simulink model "navigation_filter"  (R2024b)
settings: Solver=FixedStepAuto  StartTime=0.0  StopTime=200.0  FixedStep=ST  RelTol=1e-3
values from neighbouring files (symbols this model uses):
  bias_gyro = [0.02 0.01 0.007]    [sensors.m]    (also in sensors_2.m = [0.2 0.1 0])
  dt = ST    (= 0.01)    [WP_gen.m]
  freq_acc = 50    [sensors.m]    (also in sensors_2.m)
  freq_gyro = 10    [sensors.m]    (also in sensors_2.m)
  freq_UWB = freq_gyro    (= 10)    [sensors.m]    (also in sensors_2.m)
  g = 9.81    [trajectory_gen_cartesian.m]
  N_bases = size(P_bases_ned, 1)    [sensors.m]    (also in sensors_2.m)
  pos_ned = [pos_ned_n pos_ned_e pos_ned_d]    [WP_gen.m]    (also in trajectory_gen_cartesian.m = pos_n_filt)
  Q = 100*diag([q_pos_1, q_pos_2, q_pos_3, q_vel_1, q_vel_2, q_vel_3, q_acc_1,q_acc_2,q_acc_3, q_quat_1, q_quat_2, q_quat_3, q_quat_4, q_omega_1, q_omega_2, q_omega_3, q_bias_1, q_bias_2, q_bias_3])    [sensors.m]    (also in sensors_2.m)
  Q_att = 100*diag([q_roll, q_pitch, q_yaw, q_omega_1, q_omega_2, q_omega_3, q_bias_1, q_bias_2, q_bias_3])    [sensors_2.m]
  quat_c_b = compact(quat_b)    [trajectory_gen_cartesian.m]
  sensor_covariances = [UWB_cov, ACC_cov, MAG_cov, GYRO_cov]    [sensors.m]    (also in sensors_2.m)
  ST = 1/100    (= 0.01)    [WP_gen.m]
  std_dev_accx = 0.02    [sensors.m]    (also in sensors_2.m = 0.01)
  std_dev_accy = 0.02    [sensors.m]    (also in sensors_2.m = 0.01)
  std_dev_accz = 0.02    [sensors.m]    (also in sensors_2.m = 0.01)
  std_dev_gyro1 = 1e-7    (= 1e-07)    [sensors.m]    (also in sensors_2.m = 3e-06)
  std_dev_gyro2 = 1e-7    (= 1e-07)    [sensors.m]    (also in sensors_2.m = 3e-06)
  std_dev_gyro3 = 1e-7    (= 1e-07)    [sensors.m]    (also in sensors_2.m = 3e-06)
  std_dev_magx = 0.03    [sensors.m]    (also in sensors_2.m)
  std_dev_magy = 0.03    [sensors.m]    (also in sensors_2.m)
  std_dev_magz = 0.03    [sensors.m]    (also in sensors_2.m)
  std_dev_UWB1 = 1e-6    (= 1e-06)    [sensors.m]    (also in sensors_2.m)
  Tf = ST    [sensors.m]    (also in sensors_2.m)
  vel_n = vel_n_filt    [trajectory_gen_cartesian.m]
undefined symbols (not defined in the file or in its folder): DiscIntNeverNeededParam
libraries: cstblocks x8, simulink x3, aerolibutil x2
(part 1 of 2)
settings Model: Creator=wolfl  LastModifiedBy=wolfl

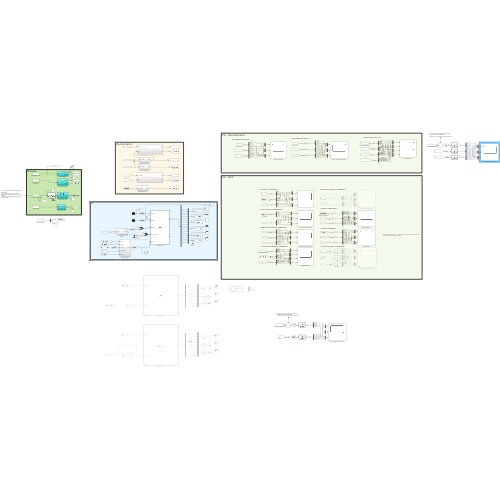
[thumbnail: Simulink's stored preview of the top-level diagram]
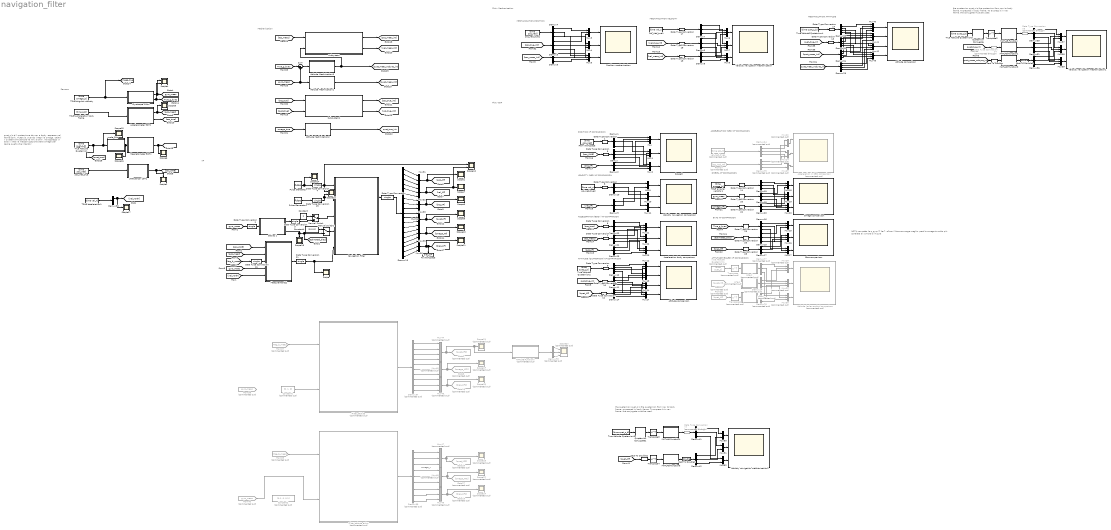
== system navigation_filter ==
  note: omega_x
  note: the quaternion quat_c is the quaternion from nav to
      | body frame, expressed in body frame.
      | To express it in nav frame, the conjugate must be used.
  note: quat_c_b è il quaternione da nav a body, espresso nel frame body.
      | Tuttavia, quando integri la omega, ottieni il quaternione sempre da nav a body, ma espresso in body!!!
      | Vedi la meccanizzazione della omega per capire quello che intendo!
  note: NOTA: se metto le q_gyro = 1e-7, allora il bias converge meglio, però la omega
      | è molto più correlata al rumore di misura
  note: Plot - EKF
  note: KF
  note: Mechanization
  note: Sensors
  note: Plot - Mechanization
  note: MECHANIZATION POSITION
  note: MECHANIZATION VELOCITY
  note: ATTUTUDE (EULER) KF COMPARISON
  note: ATTITUDE (QUATERNION) KF COMPARISON
  note: OMEGA KF COMPARISON
  note: ACCELERATION (BODY) KF COMPARISON
  note: VELOCITY (NED) KF COMPARISON
  note: POSITION KF COMPARISON
  note: BYAS KF COMPARISON
  note: ACCELERATION (NED) KF COMPARISON
  note: MECHANIZATION ATTITUDE
  note: the quaternion quat_c is the quaternion from nav to
      | body frame, expressed in body frame.
      | To express it in nav frame, the conjugate must be used.
  Acceleration body comparison : Scope  NumInputPorts=3
  Acceleration in NED comparison : Scope  Commented=on  NumInputPorts=3
  Accelerometer 50Hz : Subsystem
  Attitude (euler angles) comparison : Scope  Commented=on  NumInputPorts=3
  Attitude Mechnization1 : Subsystem
  Attitude Mechnization2 : Subsystem
  Attitude Mechnization3 : Subsystem
  "Attitude comparison " : Scope  NumInputPorts=4
  "Attitude comparison " : Scope  NumInputPorts=4
  Bias comparison : Scope  NumInputPorts=3
  Cast To Double{,1..3} (4 alike) : DataTypeConversion  OutDataTypeStr=double  SaturateOnIntegerOverflow=off  RndMeth=Floor
  Constant : Constant
  Constant1 : Constant  Commented=on  Value=[0, 1, 0]
  Constant2 : Constant  Commented=on  Value=[0.1, 0, 0.1]
  Constant4 : Constant  Value=[0 0 0]
  Data Type Conversion{,1..23,26,28} (26 alike) : DataTypeConversion  OutDataTypeStr=single  SaturateOnIntegerOverflow=off  RndMeth=Floor
  Data Type Conversion24 : DataTypeConversion  Commented=through  OutDataTypeStr=single  SaturateOnIntegerOverflow=off  RndMeth=Floor
  Data Type Conversion25 : DataTypeConversion  Commented=through  OutDataTypeStr=single  SaturateOnIntegerOverflow=off  RndMeth=Floor
  Data Type Conversion27 : DataTypeConversion  Commented=through  OutDataTypeStr=single  SaturateOnIntegerOverflow=off  RndMeth=Floor
  Demux{,1..10,15..23,30..31,35..36,41..42} (26 alike) : Demux  Outputs=3
  Demux{11..12,14,29,32..34} (7 alike) : Demux
  Demux13 : Demux  Outputs=19
  Demux{24..28,38} (6 alike) : Demux  Commented=on  Outputs=3
  Demux37 : Demux  Commented=on  Outputs=10
  Demux39 : Demux  Commented=on  Outputs=9
  Filter_attitute : MATLAB Function  Commented=on  TreatAsAtomicUnit=on
  Filter_attitute_euler : MATLAB Function  Commented=on  TreatAsAtomicUnit=on
  From Workspace : FromWorkspace  VariableName=[time pos_ned]
  From27 : From  Commented=on  GotoTag=acc_ned_KF
  From28 : From  Commented=on  GotoTag=quat_KF
  From29 : From  Commented=on  GotoTag=quat_int
  From37 : From  Commented=on  GotoTag=Mag_b_meas
  From38 : From  Commented=on  GotoTag=gyro_meas
  From39 : From  Commented=on  GotoTag=Mag_b_meas
  From40 : From  Commented=on  GotoTag=gyro_meas
  Goto13 : Goto  Commented=on  GotoTag=bias_KF2
  Goto16 : Goto  Commented=on  GotoTag=bias_KF2
  Goto2 : Goto  Commented=on  GotoTag=quat_KF2
  Goto26 : Goto  Commented=on  GotoTag=quat_KF2
  Goto27 : Goto  Commented=on  GotoTag=omega_KF2
  Goto3 : Goto  Commented=on  GotoTag=omega_KF2
  Gyroscope 10Hz : Subsystem
  MATLAB Function : MATLAB Function  TreatAsAtomicUnit=on
  MATLAB Function1 : MATLAB Function  TreatAsAtomicUnit=on
  MATLAB Function2 : MATLAB Function  Commented=on  TreatAsAtomicUnit=on
  MATLAB Function3 : MATLAB Function  TreatAsAtomicUnit=on
  MATLAB Function4 : MATLAB Function  TreatAsAtomicUnit=on
  MATLAB Function6 : MATLAB Function  TreatAsAtomicUnit=on
  Magnetometer 50Hz : Subsystem
  Manual Switch : ManualSwitch
  Manual Switch1 : ManualSwitch
  Measurements2 : Subsystem
  Mux{,1..8,12..23,27,31..33,35..39} (30 alike) : Mux  Inputs=3
  Mux{9..11,50..52} (6 alike) : Mux  Inputs=2
  Mux24 : Mux  Commented=on  Inputs=2
  Mux25 : Mux  Commented=on  Inputs=2
  Mux26 : Mux  Commented=on  Inputs=2
  Mux{28..30,45..49} (8 alike) : Mux  Commented=on  Inputs=3
  Mux{34,40..43} (5 alike) : Mux
  Mux44 : Mux  Commented=on
  Navigation Filter : MATLAB Function  TreatAsAtomicUnit=on
  Omega comparison : Scope  NumInputPorts=3
  Position mechanization : Scope  NumInputPorts=3
  Pulse Generator : DiscretePulseGenerator  PulseType=Time based  Period=0.1  PulseWidth=10  SampleTime=dt
  Pulse Generator1 : DiscretePulseGenerator  PulseType=Time based  Period=1/50  PulseWidth=50  SampleTime=dt
  Quaternion Conjugate : aerolibutil/Quaternion Conjugate
  Quaternion Conjugate1 : aerolibutil/Quaternion Conjugate
  Scope{,1..2,5..11,14..18} (15 alike) : Scope
  Scope12 : Scope  NumInputPorts=2
  Scope13 : Scope  NumInputPorts=2
  Scope{19..21,23..25} (6 alike) : Scope  Commented=on
  Scope22 : Scope  Commented=on  NumInputPorts=3
  Scope3 : Scope  NumInputPorts=3
  Scope4 : Scope  NumInputPorts=2
  Subsystem : Subsystem
  Subsystem1 : Subsystem
  Sum : Sum  Inputs=|-+
  TRUE acceleration body frame : FromWorkspace  VariableName=[time acc]  SampleTime=ST
  TRUE acceleration1 : FromWorkspace  VariableName=[time vel_n]  SampleTime=ST
  TRUE angular velocity : FromWorkspace  VariableName=[time omega_b]  SampleTime=ST
  TRUE angular velocity1 : FromWorkspace  VariableName=[time omega_b]  SampleTime=ST
  To Workspace : ToWorkspace  VariableName=bias_KF  SaveFormat=Timeseries  SampleTime=-1
  Transpose : Math  Commented=on  Operator=transpose
  Transpose1 : Math  Commented=on  Operator=transpose
  Transpose2 : Math  Operator=transpose
  Transpose3 : Math  Operator=transpose
  Transpose4 : Math  Operator=transpose
  True Attitude Quaternion{,2..5} (5 alike) : FromWorkspace  VariableName=[time quat_c_b]  SampleTime=ST
  True Attitude Quaternion1 : FromWorkspace  Commented=on  VariableName=[time quat_c]  SampleTime=ST
  UWB sensor 10Hz : Subsystem
  Velocity navigation comparison : Scope  NumInputPorts=3
  Velocity navigation mechanization : Scope  NumInputPorts=3
  Velocity navigation mechanization1 : Scope  NumInputPorts=3
  Velocity navigation mechanization2 : Scope  NumInputPorts=3
  debias 1 : Subsystem
  make Cnb : MATLAB Function  TreatAsAtomicUnit=on
  pos_ned_true : FromWorkspace  VariableName=[time pos_ned]  SampleTime=ST
  pos_ned_true1 : FromWorkspace  VariableName=[time pos_ned]  SampleTime=ST
  q2eul : MATLAB Function  Commented=on  TreatAsAtomicUnit=on
  q2eul_ : MATLAB Function  Commented=on  TreatAsAtomicUnit=on
  q2eul__ : MATLAB Function  Commented=on  TreatAsAtomicUnit=on
  vel_ned_true1 : FromWorkspace  VariableName=[time vel_n]  SampleTime=ST
  vel_ned_true2 : FromWorkspace  VariableName=[time vel_n]  SampleTime=ST
  vel_ned_true4 : FromWorkspace  Commented=on  VariableName=[time acc_n]  SampleTime=ST
  tag scope: True_g_byas=global, gyro_meas=global, omega_true=global, quat_true_int=global
  wires:
  Gyroscope 10Hz/1(omega_meas) -> Scope4/1, [gyro_meas]
  True Attitude Quaternion/1 -> Scope15/1, make Cnb/1(Q_NB), [quat_true]
  Magnetometer 50Hz/1(mag_b_meas) -> Scope6/1, [Mag_b_meas]
  Gyroscope 10Hz/2(True Byas) -> Scope4/2, [True_g_byas]
  make Cnb/1(mag_b) -> Scope16/1, Magnetometer 50Hz/1(mag_b_true)
  pos_ned_true/1 -> UWB sensor 10Hz/1(pos_ned)
  Accelerometer 50Hz/1(acc_meas) -> Scope5/1, [acc_meas]
  Accelerometer 50Hz/2(acc_true) -> [acc_true]
  [gyro_meas] -> Data Type Conversion2/1
  Data Type Conversion2/1 -> debias 1/1(omega)
  debias 1/1(flag_init) -> Data Type Conversion3/1
  Data Type Conversion3/1 -> Manual Switch/2
  Pulse Generator/1 -> Scope14/1, Data Type Conversion4/1
  Data Type Conversion4/1 -> Navigation Filter/1(flag10Hz), Scope12/1, Scope13/1
  Pulse Generator1/1 -> Data Type Conversion15/1
  Data Type Conversion15/1 -> Navigation Filter/2(flag50Hz), Scope13/2
  Data Type Conversion21/1 -> Scope/1, Navigation Filter/5(measure)
  [pos_UWB] -> Measurements2/1("meas pos ")
  [Mag_b_meas] -> Data Type Conversion16/1
  Data Type Conversion16/1 -> Measurements2/3(meas_mag)
  [gyro_meas] -> Measurements2/4(meas_omega_b)
  [acc_meas] -> Measurements2/2(meas_acc)
  debias 1/3(estimated biases gyro) -> Manual Switch1/2, [estimated_bias], Scope18/1
  Demux25/1 -> Mux26/2  "a_n KF"
  [vel_true_int] -> Data Type Conversion18/1  "true_int"
  Demux18/1 -> Mux18/2  "omega_x GYRO"
  Demux2/2 -> Mux1/3  "e KF"
  [acc_true] -> Data Type Conversion6/1  "f_b_y true"
  True Attitude Quaternion1/1 -> Transpose/1  "true"
  [vel_KF] -> Demux9/1  "KF"
  From27/1 -> Demux25/1  "KF"
  Demux17/1 -> Mux15/3  "b_x KF"
  Demux6/1 -> Mux6/2  "v_n true_int"
  Mux12/1 -> "Attitude comparison "/1
  Demux28/3 -> Mux30/3  "Yaw KF"
  Demux14/2 -> Mux13/3  "qx KF"
  q2eul__/1(y) -> Demux28/1
  Mux27/1 -> "Attitude comparison "/4
  Mux20/1 -> Omega comparison/3
  Mux17/1 -> Bias comparison/3
  Demux6/2 -> Mux7/2  "v_e true_int"
  [omega_KF] -> Data Type Conversion22/1  "KF"
  Demux27/2 -> Mux29/1  "Pitch true"
  Demux22/2 -> Mux22/1  "acc_true_y"
  q2eul/1(y) -> Demux27/1
  From29/1 -> q2eul_/1(u)  "int"
  Demux26/2 -> Mux29/2  "Pitch int"
  Mux26/1 -> Acceleration in NED comparison/1
  Mux10/1 -> Velocity navigation comparison/2
  [acc_KF] -> Demux23/1  "KF"
  Demux11/3 -> Mux14/2  "qy int"
  [pos_true_int] -> Demux3/1  "true_int"
  Mux2/1 -> Scope3/3
  [pos_meas_int] -> Demux5/1  "meas_int"
  Demux4/1 -> Mux3/1  "n true"
  Demux15/3 -> Mux17/2  "b_z rem"
  Demux7/1 -> Mux6/1  "v_n true"
  Demux27/3 -> Mux30/1  "Yaw true"
  Demux25/3 -> Mux25/2  "a_d KF"
  Mux30/1 -> Attitude (euler angles) comparison/3
  Demux1/3 -> Mux2/1  "d true"
  Demux10/3 -> Mux11/1  "v_d true"
  Demux1/2 -> Mux1/1  "e true"
  Demux12/2 -> Mux13/1  "qx true"
  Demux27/1 -> Mux28/1  "Roll true"
  Demux14/3 -> Mux14/3  "qy KF"
  Demux20/2 -> Mux19/3  "omega_y KF"
  Demux19/3 -> Mux20/1  "omega_z true"
  Demux2/3 -> Mux2/3  "d KF"
  Demux5/1 -> Mux3/3  "n meas_int"
  Mux14/1 -> "Attitude comparison "/3
  Mux6/1 -> Velocity navigation mechanization/1
  Demux14/4 -> Mux27/3  "qz KF"
  Demux7/2 -> Mux7/1  "v_e true"
  Mux25/1 -> Acceleration in NED comparison/3
  Demux9/3 -> Mux11/2  "v_d KF"
  [vel_meas_int] -> Data Type Conversion19/1  "meas_int"
  [bias_KF] -> Data Type Conversion28/1  "KF"
  Mux15/1 -> Bias comparison/1
  Demux28/1 -> Mux28/3  "Roll KF"
  Demux16/1 -> Mux15/1  "b_x true"
  Demux2/1 -> Mux/3  "n KF"
  Demux24/2 -> Mux24/1  "a_e true"
  [acc_meas] -> Data Type Conversion7/1  "ACC"
  Demux22/3 -> Mux23/1  "acc_true_z"
  Demux19/1 -> Mux18/1  "omega_x true"
  [pos_UWB] -> Data Type Conversion5/1  "UWB"
  From28/1 -> Transpose1/1  "KF"
  Demux5/2 -> Mux4/3  "e meas_int"
  Demux12/3 -> Mux14/1  "qy true"
  Mux22/1 -> Acceleration body comparison/2
  Demux23/2 -> Mux22/3  "acc_y KF"
  Demux23/1 -> Mux21/3  "acc_x KF"
  Demux18/2 -> Mux19/2  "omega_y GYRO"
  Demux28/2 -> Mux29/3  "Pitch KF"
  pos_ned_true1/1 -> Demux4/1  "true"
  Demux11/4 -> Mux27/2  "qz int"
  Demux12/4 -> Mux27/1  "qz true"
  Demux17/2 -> Mux16/3  "b_y KF"
  Demux8/3 -> Mux8/3  "v_d meas_int"
  Demux21/1 -> Mux21/2  "acc_meas_x"
  Demux16/3 -> Mux17/1  "b_z true"
  Demux19/2 -> Mux19/1  "omega_y true"
  Demux8/2 -> Mux7/3  "v_e meas_int"
  [pos_KF] -> Demux2/1  "KF"
  Demux8/1 -> Mux6/3  "v_n meas_int"
  Demux15/1 -> Mux15/2  "b_x rem"
  Demux12/1 -> Mux12/1  "qw true"
  Demux11/1 -> Mux12/2  "qw int"
  Mux8/1 -> Velocity navigation mechanization/3
  Demux3/3 -> Mux5/2  "d true_int"
  Mux7/1 -> Velocity navigation mechanization/2
  Demux21/2 -> Mux22/2  "acc_meas_y"
  Demux5/3 -> Mux5/3  "d meas_int"
  Mux16/1 -> Bias comparison/2
  Demux15/2 -> Mux16/2  "b_y rem"
  Demux/1 -> Mux/2  "n UWB"
  Demux3/2 -> Mux4/2  "e true_int"
  Demux16/2 -> Mux16/1  "b_y true"
  Mux24/1 -> Acceleration in NED comparison/2
  Demux25/2 -> Mux24/2  "a_e KF"
  Demux7/3 -> Mux8/1  "v_d true"
  Demux20/1 -> Mux18/3  "omega_x KF"
  Mux28/1 -> Attitude (euler angles) comparison/1
  Mux1/1 -> Scope3/2
  Demux23/3 -> Mux23/3  "acc_z KF"
  q2eul_/1(y) -> Demux26/1
  [quat_KF] -> Data Type Conversion12/1  "KF"
  Mux5/1 -> Position mechanization/3
  Demux14/1 -> Mux12/3  "qw KF"
  vel_ned_true4/1 -> Demux24/1  "true"
  Demux22/1 -> Mux21/1  "acc_true_x"
  Demux24/1 -> Mux26/1  "a_n true"
  Demux10/1 -> Mux9/1  "v_n true"
  Transpose/1 -> q2eul/1(u)
  Demux4/2 -> Mux4/1  "e true"
  Demux24/3 -> Mux25/1  "a_d true"
  Demux9/1 -> Mux9/2  "v_n KF"
  Demux26/1 -> Mux28/2  "Roll int"
  Demux11/2 -> Mux13/2  "qw int"
  Demux/3 -> Mux2/2  "d UWB"
  [estimated_bias] -> Data Type Conversion26/1  "removed"
  Mux18/1 -> Omega comparison/1
  Demux3/1 -> Mux3/2  "n true_int"
  Demux9/2 -> Mux10/2  "v_e KF"
  Mux21/1 -> Acceleration body comparison/1
  vel_ned_true1/1 -> Data Type Conversion17/1  "true"
  [True_g_byas] -> Data Type Conversion23/1  "true"
  vel_ned_true2/1 -> Data Type Conversion8/1  "true"
  Demux21/3 -> Mux23/2  "acc_meas_z"
  Demux6/3 -> Mux8/2  "v_d true_int"
  Mux11/1 -> Velocity navigation comparison/3
  Mux23/1 -> Acceleration body comparison/3
  Demux20/3 -> Mux20/3  "omega_z KF"
  Mux/1 -> Scope3/1
  Mux3/1 -> Position mechanization/1
  Mux4/1 -> Position mechanization/2
  TRUE angular velocity1/1 -> Data Type Conversion11/1  "true"
  Demux/2 -> Mux1/2  "e UWB"
  Mux9/1 -> Velocity navigation comparison/1
  Demux26/3 -> Mux30/2  "Yaw int"
  Mux29/1 -> Attitude (euler angles) comparison/2
  Demux10/2 -> Mux10/1  "v_e true"
  Demux1/1 -> Mux/1  "n true"
  Mux13/1 -> "Attitude comparison "/2
  Transpose1/1 -> q2eul__/1(u)
  Demux17/3 -> Mux17/3  "b_z KF"
  Demux18/3 -> Mux20/2  "omega_z GYRO"
  Demux4/3 -> Mux5/1  "d true"
  Mux19/1 -> Omega comparison/2
  Navigation Filter/1(xout) -> Data Type Conversion/1
  Demux13/1 -> Mux31/1
  Demux13/2 -> Mux31/2
  Demux13/3 -> Mux31/3
  Mux31/1 -> Scope1/1, [pos_KF]
  Demux13/4 -> Mux32/1
  Demux13/5 -> Mux32/2
  Demux13/6 -> Mux32/3
  Mux32/1 -> Scope12/2, Scope7/1, [vel_KF]
  Demux13/9 -> Mux33/3
  Demux13/7 -> Mux33/1
  Demux13/8 -> Mux33/2
  Mux33/1 -> Scope8/1, [acc_KF]
  Demux13/12 -> Mux34/3
  Demux13/10 -> Mux34/1
  Demux13/11 -> Mux34/2
  Mux34/1 -> Scope9/1, [quat_KF]
  Demux13/13 -> Mux34/4
  Demux13/16 -> Mux35/3
  Demux13/14 -> Mux35/1
  Demux13/15 -> Mux35/2
  Mux35/1 -> Scope10/1, [omega_KF]
  Demux13/19 -> Mux36/3
  Demux13/17 -> Mux36/1
  Demux13/18 -> Mux36/2
  Mux36/1 -> [bias_KF], To Workspace/1, Scope11/1
  From Workspace/1 -> Data Type Conversion1/1
  Data Type Conversion/1 -> Demux13/1
  Data Type Conversion1/1 -> Demux1/1
  Data Type Conversion5/1 -> Demux/1
  Data Type Conversion6/1 -> Demux22/1
  Data Type Conversion7/1 -> Demux21/1
  Data Type Conversion8/1 -> Demux10/1
  Data Type Conversion9/1 -> Demux12/1
  Data Type Conversion10/1 -> Demux11/1
  True Attitude Quaternion2/1 -> Data Type Conversion9/1  "true"
  Data Type Conversion11/1 -> Demux19/1
  [acc_meas] -> Subsystem/1(acc_body)
  [gyro_meas] -> Sum/2, Attitude Mechnization1/1(omega_meas)
  Attitude Mechnization1/1(q_NB) -> [quat_meas_int]
  Subsystem/1(pos) -> [pos_meas_int]
  Subsystem/2(vel) -> [vel_meas_int]
  Subsystem1/1(pos) -> [pos_true_int]
  Subsystem1/2(vel) -> [vel_true_int]
  Attitude Mechnization2/1(q_NB) -> [quat_true_int]
  [acc_true] -> Subsystem1/1(acc_body)
  [omega_true] -> Attitude Mechnization2/1(omega_meas)
  Mux43/1 -> "Attitude comparison "/4
  Demux34/4 -> Mux43/3  "qz meas int"
  Demux33/2 -> Mux41/1  "qx true"
  Demux32/2 -> Mux41/2  "qw int"
  Demux33/4 -> Mux43/1  "qz true"
  Demux32/3 -> Mux42/2  "qy int"
  Demux34/1 -> Mux40/3  "qw meas int"
  Demux33/3 -> Mux42/1  "qy true"
  True Attitude Quaternion4/1 -> Data Type Conversion14/1  "true"
  Mux42/1 -> "Attitude comparison "/3
  Data Type Conversion13/1 -> Demux32/1
  Mux40/1 -> "Attitude comparison "/1
  Demux32/4 -> Mux43/2  "qz int"
  Demux34/2 -> Mux41/3  "qx meas int"
  Demux33/1 -> Mux40/1  "qw true"
  Demux34/3 -> Mux42/3  "qy meas int"
  Data Type Conversion14/1 -> Demux33/1
  Demux32/1 -> Mux40/2  "qw int"
  Mux41/1 -> "Attitude comparison "/2
  [quat_true_int] -> Data Type Conversion13/1  "true_int"
  [quat_meas_int] -> Demux34/1  "meas_int"
  [True_g_byas] -> Sum/1
  Attitude Mechnization3/1(q_NB) -> Subsystem/2(q_NB), [quat_meas_nobyas_int]
  Sum/1 -> Attitude Mechnization3/1(omega_meas)
  Demux29/1 -> Mux40/4  "qw meas nobyas int"
  Demux29/2 -> Mux41/4  "qx meas nobyas int"
  Demux29/3 -> Mux42/4  "qy meas nobyas int"
  [quat_meas_nobyas_int] -> Demux29/1  "meas_int"
  Demux29/4 -> Mux43/4  "qz meas nobyas int"
  Data Type Conversion17/1 -> Demux7/1
  Data Type Conversion18/1 -> Demux6/1
  Data Type Conversion19/1 -> Demux8/1
  TRUE acceleration1/1 -> Demux30/1
  Demux30/1 -> Scope17/1, [vel_north]
  [vel_north] -> Measurements2/5(meas_vel_n)
  Measurements2/1(KF meas) -> Data Type Conversion21/1
  UWB sensor 10Hz/1("UWB pos ") -> Scope2/1, [pos_UWB]  "true"
  Data Type Conversion26/1 -> Demux15/1
  Data Type Conversion28/1 -> Demux17/1
  [quat_true_int] -> Data Type Conversion10/1  "true_int"
  Demux36/2 -> Mux38/3  "att_meas_int"
  MATLAB Function1/1(euler) -> Demux31/1
  Demux31/3 -> Mux39/2  "att_true_int"
  Data Type Conversion25/1 -> Demux35/1
  Demux35/2 -> Mux38/1  "att_true"
  Transpose2/1 -> MATLAB Function/1(q)  "true"
  MATLAB Function3/1(euler) -> Cast To Double1/1
  Cast To Double/1 -> MATLAB Function3/1(q)
  Demux36/1 -> Mux37/3  "att_meas_int"
  Mux39/1 -> Velocity navigation mechanization1/3
  [quat_meas_nobyas_int] -> Cast To Double/1  "meas_int"
  True Attitude Quaternion5/1 -> Quaternion Conjugate/1  "true"
  Demux36/3 -> Mux39/3  "att_meas_int"
  Mux38/1 -> Velocity navigation mechanization1/2
  [quat_true_int] -> Data Type Conversion24/1  "true_int"
  Demux31/2 -> Mux38/2  "att_ true_int"
  MATLAB Function/1(euler) -> Data Type Conversion25/1
  Data Type Conversion24/1 -> MATLAB Function1/1(q)
  Cast To Double1/1 -> Demux36/1
  Mux37/1 -> Velocity navigation mechanization1/1
  Demux31/1 -> Mux37/2  "att_true_int"
  Demux35/3 -> Mux39/1  "att_true"
  Demux35/1 -> Mux37/1  "att_true"
  Quaternion Conjugate/1 -> Transpose2/1
  Manual Switch/1 -> Navigation Filter/3(flagINITOK)
  Constant/1 -> Manual Switch/1
  Manual Switch1/1 -> Navigation Filter/4(bias_gyro_removed)
  Constant4/1 -> Manual Switch1/1
  From37/1 -> Filter_attitute/1(mag_meas)
  Constant1/1 -> Filter_attitute/2(omega_meas)
  Filter_attitute/1(x_out) -> Demux37/1
  Demux37/1 -> Mux44/1
  Demux37/2 -> Mux44/2
  Demux37/3 -> Mux44/3
  Demux37/4 -> Mux44/4
  Demux37/5 -> Mux45/1  "omega_x"
  Demux37/6 -> Mux45/2  "omega_y"
  Demux37/7 -> Mux45/3  "omega_z"
  Demux37/8 -> Mux46/1
  Demux37/9 -> Mux46/2
  Demux37/10 -> Mux46/3
  Mux45/1 -> Scope19/1, Goto3/1
  Mux44/1 -> Goto2/1, MATLAB Function2/1(q_c), Scope21/1
  Mux46/1 -> Goto13/1, Scope20/1
  MATLAB Function2/1(eulerAngles) -> Demux38/1
  Demux38/1 -> Scope22/1  "yaw"
  Demux38/2 -> Scope22/2  "pitch"
  Demux38/3 -> Scope22/3  "roll"
  Demux39/7 -> Mux49/1  "bias_x"
  Demux39/8 -> Mux49/2  "bias_y"
  From39/1 -> Filter_attitute_euler/1(mag_meas)
  From40/1 -> Filter_attitute_euler/2(omega_meas)
  Filter_attitute_euler/1(x_out) -> Demux39/1
  Mux49/1 -> Goto16/1, Scope24/1
  Demux39/6 -> Mux48/3  "omega_z"
  Mux47/1 -> Goto26/1, Scope25/1
  Mux48/1 -> Goto27/1, Scope23/1
  Demux39/1 -> Mux47/1  "roll"
  Demux39/5 -> Mux48/2  "omega_y"
  Demux39/4 -> Mux48/1
  Demux39/9 -> Mux49/3  "bias_z"
  Demux39/3 -> Mux47/3  "yaw"
  Demux39/2 -> Mux47/2  "pitch"
  TRUE acceleration body frame/1 -> Accelerometer 50Hz/1(acc_b)
  TRUE angular velocity/1 -> [omega_true], Gyroscope 10Hz/1(pqr_true)
  Demux41/3 -> Mux52/1  "att_true"
  Mux51/1 -> Velocity navigation mechanization2/2
  Data Type Conversion27/1 -> Demux41/1
  Demux41/1 -> Mux50/1  "att_true"
  MATLAB Function4/1(euler) -> Data Type Conversion27/1
  Demux42/3 -> Mux52/2  "quat_KF_yaw"
  [quat_KF] -> Cast To Double2/1  "meas_int"
  MATLAB Function6/1(rpy) -> Cast To Double3/1
  Mux50/1 -> Velocity navigation mechanization2/1
  Demux42/2 -> Mux51/2  "quat_KF_pitchl"
  Demux41/2 -> Mux51/1  "att_true"
  Transpose3/1 -> MATLAB Function4/1(q)  "true"
  Cast To Double3/1 -> Demux42/1
  Demux42/1 -> Mux50/2  "quat_KF_roll"
  Mux52/1 -> Velocity navigation mechanization2/3
  Cast To Double2/1 -> Transpose4/1
  Quaternion Conjugate1/1 -> Transpose3/1
  True Attitude Quaternion3/1 -> Quaternion Conjugate1/1  "true"
  Transpose4/1 -> MATLAB Function6/1(q)  "true"
  [quat_true] -> Subsystem1/2(q_NB)
  [gyro_meas] -> Data Type Conversion20/1  "GYRO"
  Data Type Conversion20/1 -> Demux18/1
  Data Type Conversion22/1 -> Demux20/1
  Data Type Conversion23/1 -> Demux16/1
  Data Type Conversion12/1 -> Demux14/1

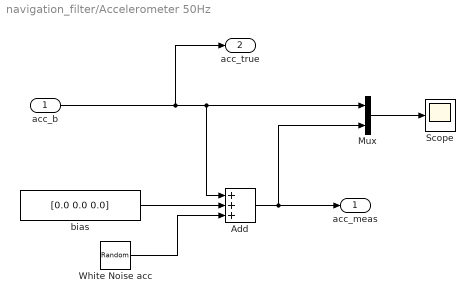
== system navigation_filter/Accelerometer 50Hz ==
  acc_b : Inport
  Add : Sum  Inputs=+++
  Mux : Mux  Inputs=2
  Scope : Scope
  White Noise acc : RandomNumber  DisableCoverage=on  Mean=[0 0 0 ]  Variance=[std_dev_accx^2, std_dev_accy^2, std_dev_accz^2]  Seed=[1, 2, 3]  SampleTime=1/freq_acc
  bias : Constant  Value=[0.0 0.0 0.0]
  acc_meas : Outport
  acc_true : Outport  Port=2
  wires:
  acc_b/1 -> acc_true/1, Add/1, Mux/1
  White Noise acc/1 -> Add/3
  Mux/1 -> Scope/1
  Add/1 -> Mux/2, acc_meas/1
  bias/1 -> Add/2

== system navigation_filter/Attitude Mechnization1 ==
  omega_meas : Inport
  Delay : Delay  DelayLength=1  InitialCondition=quat_c_b(1,:)
  quaternion update : MATLAB Function  TreatAsAtomicUnit=on
  q_NB : Outport
  wires:
  omega_meas/1 -> quaternion update/1(omega_meas)
  quaternion update/1(q_NB_p) -> q_NB/1, Delay/1
  Delay/1 -> quaternion update/2(q_NB)

== system navigation_filter/Attitude Mechnization2 ==
  omega_meas : Inport
  Delay : Delay  DelayLength=1  InitialCondition=quat_c_b(1,:)
  quaternion update : MATLAB Function  TreatAsAtomicUnit=on
  q_NB : Outport
  wires:
  omega_meas/1 -> quaternion update/1(omega_meas)
  quaternion update/1(q_NB_p) -> q_NB/1, Delay/1
  Delay/1 -> quaternion update/2(q_NB)

== system navigation_filter/Attitude Mechnization3 ==
  omega_meas : Inport
  Delay : Delay  DelayLength=1  InitialCondition=quat_c_b(1,:)
  quaternion update : MATLAB Function  TreatAsAtomicUnit=on
  q_NB : Outport
  wires:
  omega_meas/1 -> quaternion update/1(omega_meas)
  quaternion update/1(q_NB_p) -> q_NB/1, Delay/1
  Delay/1 -> quaternion update/2(q_NB)

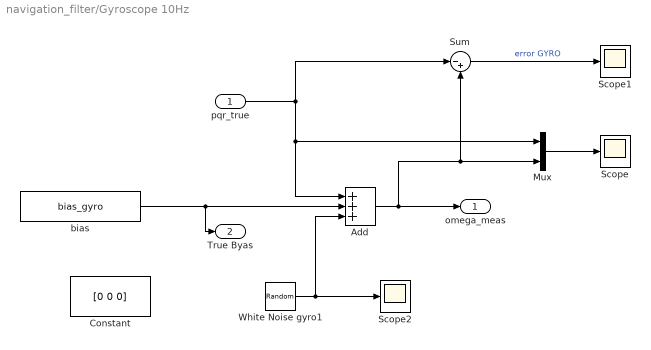
== system navigation_filter/Gyroscope 10Hz ==
  pqr_true : Inport
  Add : Sum  Inputs=+++
  Constant : Constant  Value=[0 0 0]
  Mux : Mux  Inputs=2
  Scope : Scope
  Scope1 : Scope
  Scope2 : Scope
  Sum : Sum  Inputs=|-+
  White Noise gyro1 : RandomNumber  DisableCoverage=on  Mean=[0 0 0]  Variance=[std_dev_gyro1,std_dev_gyro2,std_dev_gyro3]  Seed=[4 5 6]  SampleTime=1/freq_gyro
  bias : Constant  Value=bias_gyro  SampleTime=ST
  omega_meas : Outport
  True Byas : Outport  Port=2
  wires:
  Mux/1 -> Scope/1
  pqr_true/1 -> Mux/1, Add/1, Sum/1
  White Noise gyro1/1 -> Add/3, Scope2/1
  Add/1 -> Sum/2, Mux/2, omega_meas/1
  Sum/1 -> Scope1/1  "error GYRO"
  bias/1 -> True Byas/1, Add/2

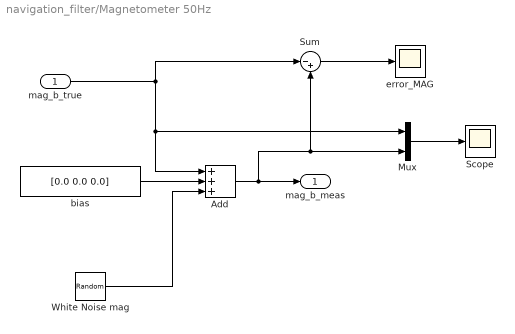
== system navigation_filter/Magnetometer 50Hz ==
  mag_b_true : Inport
  Add : Sum  Inputs=+++
  Mux : Mux  Inputs=2
  Scope : Scope
  Sum : Sum  Inputs=|-+
  White Noise mag : RandomNumber  DisableCoverage=on  Mean=[0 0 0]  Variance=[std_dev_magx^2, std_dev_magy^2, std_dev_magz^2]  Seed=[7 8 9]  SampleTime=Tf
  bias : Constant  Value=[0.0 0.0 0.0]
  error_MAG : Scope
  mag_b_meas : Outport
  wires:
  Add/1 -> Sum/2, Mux/2, mag_b_meas/1
  mag_b_true/1 -> Mux/1, Add/1, Sum/1
  Mux/1 -> Scope/1
  bias/1 -> Add/2
  White Noise mag/1 -> Add/3
  Sum/1 -> error_MAG/1

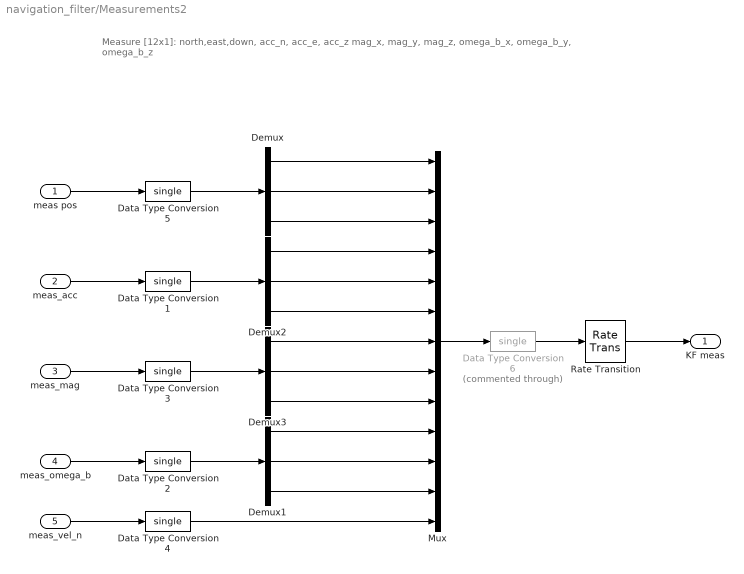
== system navigation_filter/Measurements2 ==
  note: Measure [12x1]: north,east,down,
      | acc_n, acc_e, acc_z
      | mag_x, mag_y, mag_z,
      | omega_b_x, omega_b_y, omega_b_z
  "meas pos " : Inport
  meas_acc : Inport  Port=2
  meas_mag : Inport  Port=3
  meas_omega_b : Inport  Port=4
  meas_vel_n : Inport  Port=5
  Data Type Conversion{1..5} (5 alike) : DataTypeConversion  OutDataTypeStr=single  SaturateOnIntegerOverflow=off  RndMeth=Floor
  Data Type Conversion6 : DataTypeConversion  Commented=through  OutDataTypeStr=single  SaturateOnIntegerOverflow=off  RndMeth=Floor
  Demux{,1..3} (4 alike) : Demux  Outputs=3
  Mux : Mux  Inputs=13
  Rate Transition : RateTransition  OutPortSampleTime=1/50
  KF meas : Outport
  wires:
  Demux1/3 -> Mux/12
  Demux1/2 -> Mux/11
  Demux1/1 -> Mux/10
  Demux3/3 -> Mux/9
  Demux3/2 -> Mux/8
  Demux3/1 -> Mux/7
  Demux2/3 -> Mux/6
  Demux2/2 -> Mux/5
  Demux2/1 -> Mux/4
  Data Type Conversion5/1 -> Demux/1
  Demux/3 -> Mux/3
  meas_acc/1 -> Data Type Conversion1/1
  meas_omega_b/1 -> Data Type Conversion2/1
  Demux/1 -> Mux/1
  Demux/2 -> Mux/2
  Data Type Conversion3/1 -> Demux3/1
  Data Type Conversion2/1 -> Demux1/1
  Data Type Conversion1/1 -> Demux2/1
  meas_mag/1 -> Data Type Conversion3/1
  Rate Transition/1 -> KF meas/1
  "meas pos "/1 -> Data Type Conversion5/1
  Data Type Conversion6/1 -> Rate Transition/1
  Mux/1 -> Data Type Conversion6/1
  meas_vel_n/1 -> Data Type Conversion4/1
  Data Type Conversion4/1 -> Mux/13

== system navigation_filter/Subsystem ==
  acc_body : Inport
  q_NB : Inport  Port=2
  Discrete-Time Integrator : DiscreteIntegrator  InitialCondition=vel_n(1,:)  SampleTime=-1  ICPrevOutput=DiscIntNeverNeededParam  ICPrevScaledInput=DiscIntNeverNeededParam
  Discrete-Time Integrator1 : DiscreteIntegrator  InitialCondition=pos_ned(1,:)  SampleTime=-1  ICPrevOutput=DiscIntNeverNeededParam  ICPrevScaledInput=DiscIntNeverNeededParam
  Matrix Multiply : Product  Multiplication=Matrix(*)
  make Cbn : MATLAB Function  TreatAsAtomicUnit=on
  pos : Outport
  vel : Outport  Port=2
  wires:
  Discrete-Time Integrator/1 -> vel/1, Discrete-Time Integrator1/1
  Discrete-Time Integrator1/1 -> pos/1
  acc_body/1 -> Matrix Multiply/2
  q_NB/1 -> make Cbn/1(q)
  make Cbn/1(R_nb) -> Matrix Multiply/1
  Matrix Multiply/1 -> Discrete-Time Integrator/1

== system navigation_filter/Subsystem1 ==
  acc_body : Inport
  q_NB : Inport  Port=2
  Discrete-Time Integrator : DiscreteIntegrator  InitialCondition=vel_n(1,:)  SampleTime=-1  ICPrevOutput=DiscIntNeverNeededParam  ICPrevScaledInput=DiscIntNeverNeededParam
  Discrete-Time Integrator1 : DiscreteIntegrator  InitialCondition=pos_ned(1,:)  SampleTime=-1  ICPrevOutput=DiscIntNeverNeededParam  ICPrevScaledInput=DiscIntNeverNeededParam
  Matrix Multiply : Product  Multiplication=Matrix(*)
  make Cbn : MATLAB Function  TreatAsAtomicUnit=on
  pos : Outport
  vel : Outport  Port=2
  wires:
  Discrete-Time Integrator/1 -> vel/1, Discrete-Time Integrator1/1
  Discrete-Time Integrator1/1 -> pos/1
  acc_body/1 -> Matrix Multiply/2
  q_NB/1 -> make Cbn/1(q)
  make Cbn/1(R_nb) -> Matrix Multiply/1
  Matrix Multiply/1 -> Discrete-Time Integrator/1

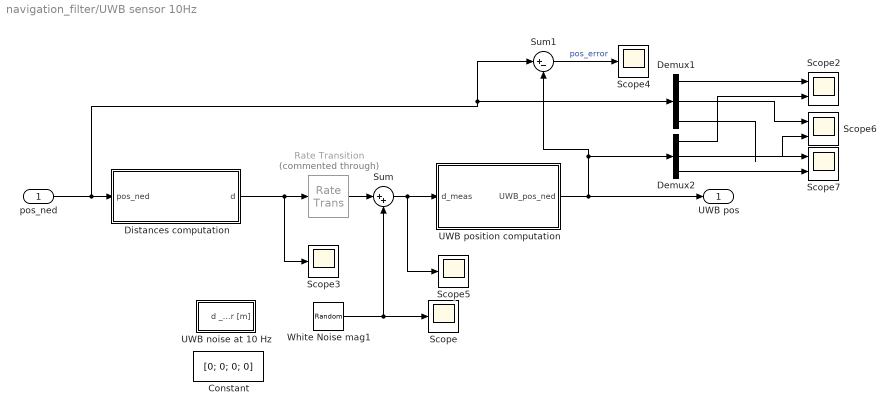
== system navigation_filter/UWB sensor 10Hz ==
  pos_ned : Inport  PortDimensions=3
  Constant : Constant  Value=[0; 0; 0; 0]
  Demux1 : Demux  Outputs=3
  Demux2 : Demux  Outputs=3
  Distances computation : MATLAB Function  TreatAsAtomicUnit=on
  Rate Transition : RateTransition  Commented=through  OutPortSampleTime=1/10
  Scope{,3..5} (4 alike) : Scope
  Scope2 : Scope  NumInputPorts=2
  Scope6 : Scope  NumInputPorts=2
  Scope7 : Scope  NumInputPorts=2
  Sum : Sum  Inputs=|++
  Sum1 : Sum  Inputs=|+-
  UWB noise at 10 Hz : Subsystem  mask{AMPd1=5, AMPd2=5, AMPd3=5, AMPd4=5, newnoise=on, seed_user=0}
      mask prompts: AMPd1 "UWB approx max error d1 [m]"; AMPd2 "UWB approx max error d2 [m]"; AMPd3 "UWB approx max error d3 [m]"; AMPd4 "UWB approx max error d4 [m]"; newnoise "new noise at each run"; seed_user "user provided seed value"
      mask init:
      | if newnoise,
      |         seedx=rand(1)*1000;
      |         seedy=rand(1)*1000;
      |         seedz=rand(1)*1000;
      |     else
      |         seedx=seed_user;
      |         seedy=seed_user+1;
      |         seedz=seed_user+2;
      |     end
      mask DialogControl ParameterGroupVar Prompt: Noise generation
  UWB position computation : MATLAB Function  TreatAsAtomicUnit=on
  White Noise mag1 : RandomNumber  DisableCoverage=on  Mean=zeros(N_bases,1)  Variance=std_dev_UWB1*ones(N_bases,1)  Seed=7:7+N_bases-1  SampleTime=1/freq_UWB
  "UWB pos " : Outport
  wires:
  pos_ned/1 -> Distances computation/1(pos_ned), Demux1/1, Sum1/1
  White Noise mag1/1 -> Scope/1, Sum/2
  Sum/1 -> Scope5/1, UWB position computation/1(d_meas)
  Distances computation/1(d) -> Rate Transition/1, Scope3/1
  Sum1/1 -> Scope4/1  "pos_error"
  Demux2/2 -> Scope6/2
  Demux1/2 -> Scope6/1
  Demux1/1 -> Scope2/1
  Demux2/1 -> Scope2/2
  Demux1/3 -> Scope7/1
  Demux2/3 -> Scope7/2
  UWB position computation/1(UWB_pos_ned) -> "UWB pos "/1, Sum1/2, Demux2/1
  Rate Transition/1 -> Sum/1

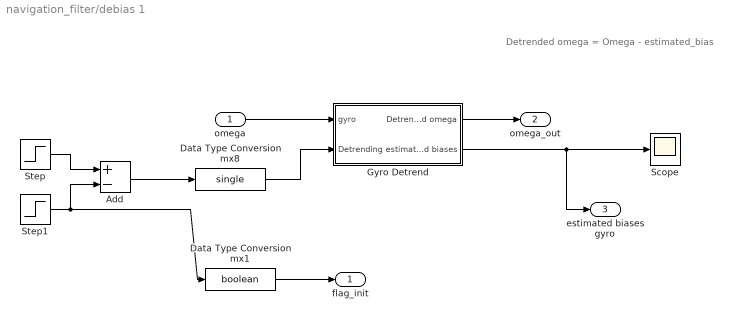
== system navigation_filter/debias 1 ==
  note: Detrended omega = Omega - estimated_bias
  omega : Inport
  Add : Sum  Inputs=+-
  Data Type Conversion mx1 : DataTypeConversion  OutDataTypeStr=boolean  RndMeth=Round
  Data Type Conversion mx8 : DataTypeConversion  OutDataTypeStr=single  RndMeth=Round
  "Gyro Detrend " : Subsystem  mask{ST2=ST}
      mask prompts: ST2 "Sample Time"
  Scope : Scope
  Step : Step  Time=0.02  SampleTime=ST
  Step1 : Step  SampleTime=ST
  flag_init : Outport
  omega_out : Outport  Port=2
  estimated biases gyro : Outport  Port=3
  wires:
  "Gyro Detrend "/2(estimated biases) -> estimated biases gyro/1, Scope/1
  Data Type Conversion mx8/1 -> "Gyro Detrend "/2(Detrending)
  Data Type Conversion mx1/1 -> flag_init/1
  "Gyro Detrend "/1(Detrended omega) -> omega_out/1
  omega/1 -> "Gyro Detrend "/1(gyro)
  Add/1 -> Data Type Conversion mx8/1
  Step1/1 -> Data Type Conversion mx1/1, Add/2
  Step/1 -> Add/1

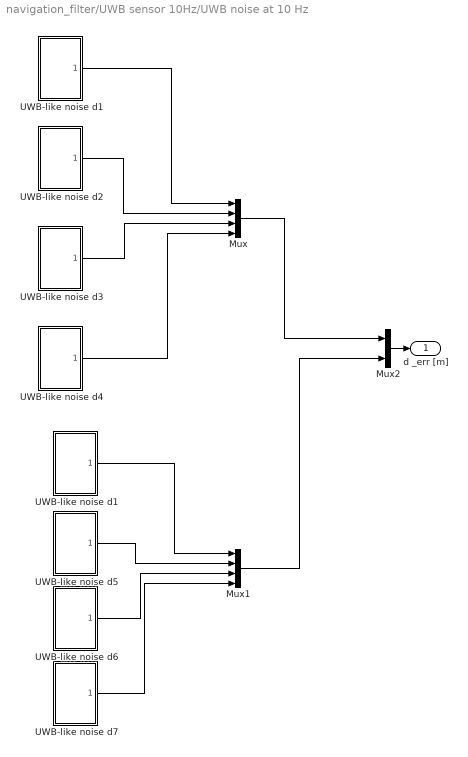
== system navigation_filter/UWB sensor 10Hz/UWB noise at 10 Hz ==
  Mux : Mux
  Mux1 : Mux
  Mux2 : Mux  Inputs=2
  UWB-like noise d1 : Subsystem
  "UWB-like noise d1 " : Subsystem
  UWB-like noise d2 : Subsystem
  UWB-like noise d3 : Subsystem
  UWB-like noise d4 : Subsystem
  UWB-like noise d5 : Subsystem
  UWB-like noise d6 : Subsystem
  UWB-like noise d7 : Subsystem
  d _err [m] : Outport
  wires:
  "UWB-like noise d1 "/1(d1_err) -> Mux/1
  Mux/1 -> Mux2/1
  UWB-like noise d2/1(d2_err) -> Mux/2
  UWB-like noise d3/1(d3_err) -> Mux/3
  UWB-like noise d4/1(d4_err) -> Mux/4
  Mux1/1 -> Mux2/2
  UWB-like noise d1/1(d4_err) -> Mux1/1
  UWB-like noise d5/1(d4_err) -> Mux1/2
  UWB-like noise d6/1(d4_err) -> Mux1/3
  UWB-like noise d7/1(d4_err) -> Mux1/4
  Mux2/1 -> d _err [m]/1

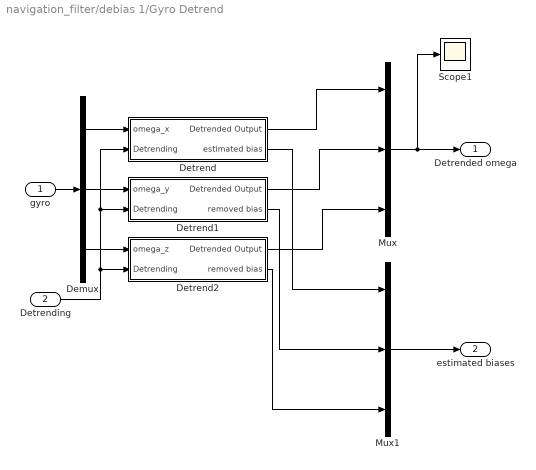
== system navigation_filter/debias 1/Gyro Detrend  ==
  gyro : Inport
  Detrending : Inport  Port=2
  Demux : Demux  Outputs=3
      settings: DisplayOption=none
  Detrend : Subsystem  mask{ST=ST2}
      mask prompts: ST "Sample Time"
  Detrend1 : Subsystem  mask{ST=ST2}
      mask prompts: ST "Sample Time"
  Detrend2 : Subsystem  mask{ST=ST2}
      mask prompts: ST "Sample Time"
  Mux : Mux  Inputs=3
  Mux1 : Mux  Inputs=3
  Scope1 : Scope
  Detrended omega : Outport
  estimated biases : Outport  Port=2
  wires:
  Detrend/2("estimated bias ") -> Mux1/1
  Detrend2/2("removed bias ") -> Mux1/3
  Detrend1/2("removed bias ") -> Mux1/2
  Mux1/1 -> estimated biases/1
  Detrend/1(Detrended Output) -> Mux/1
  Detrend1/1(Detrended Output) -> Mux/2
  Detrend2/1(Detrended Output) -> Mux/3
  Mux/1 -> Scope1/1, Detrended omega/1
  Demux/1 -> Detrend/1(omega_x)
  Demux/2 -> Detrend1/1(omega_y)
  gyro/1 -> Demux/1
  Demux/3 -> Detrend2/1(omega_z)
  Detrending/1 -> Detrend/2(Detrending), Detrend1/2(Detrending), Detrend2/2(Detrending)

== system navigation_filter/UWB sensor 10Hz/UWB noise at 10 Hz/UWB-like noise d1 ==
  Gain : Gain  Gain=0.75
  Gain1 : Gain  Gain=AMPd4
  LTI System1 : cstblocks/LTI System  sys=c2d(tf(1,[0.75 1])*tf([3000 0],[3000 1]),1/10)  IC=[]  PadeOrder=0
  Random Number : RandomNumber  Variance=0.01  Seed=13  SampleTime=1/freq_UWB
  d4_err : Outport
  wires:
  Gain1/1 -> Gain/1
  Gain/1 -> LTI System1/1
  Random Number/1 -> Gain1/1
  LTI System1/1 -> d4_err/1

== system navigation_filter/UWB sensor 10Hz/UWB noise at 10 Hz/UWB-like noise d1  ==
  Gain : Gain  Gain=0.75
  Gain1 : Gain  Gain=AMPd1
  LTI System1 : cstblocks/LTI System  sys=c2d(tf(1,[0.75 1])*tf([3000 0],[3000 1]),1/10)  IC=[]  PadeOrder=0
  Random Number : RandomNumber  Variance=0.01  Seed=10  SampleTime=1/freq_UWB
  Scope : Scope
  Scope1 : Scope
  Scope2 : Scope
  d1_err : Outport
  wires:
  Gain1/1 -> Gain/1
  Gain/1 -> Scope/1, LTI System1/1
  Random Number/1 -> Gain1/1
  LTI System1/1 -> Scope2/1, d1_err/1, Scope1/1

== system navigation_filter/UWB sensor 10Hz/UWB noise at 10 Hz/UWB-like noise d2 ==
  Gain : Gain  Gain=0.75
  Gain1 : Gain  Gain=AMPd2
  LTI System1 : cstblocks/LTI System  sys=c2d(tf(1,[0.75 1])*tf([3000 0],[3000 1]),1/10)  IC=[]  PadeOrder=0
  Random Number : RandomNumber  Variance=0.01  Seed=11  SampleTime=1/freq_UWB
  d2_err : Outport
  wires:
  Gain1/1 -> Gain/1
  Gain/1 -> LTI System1/1
  Random Number/1 -> Gain1/1
  LTI System1/1 -> d2_err/1

== system navigation_filter/UWB sensor 10Hz/UWB noise at 10 Hz/UWB-like noise d3 ==
  Gain : Gain  Gain=0.75
  Gain1 : Gain  Gain=AMPd3
  LTI System1 : cstblocks/LTI System  sys=c2d(tf(1,[0.75 1])*tf([3000 0],[3000 1]),1/10)  IC=[]  PadeOrder=0
  Random Number : RandomNumber  Variance=0.01  Seed=12  SampleTime=1/freq_UWB
  d3_err : Outport
  wires:
  Gain1/1 -> Gain/1
  Gain/1 -> LTI System1/1
  Random Number/1 -> Gain1/1
  LTI System1/1 -> d3_err/1

== system navigation_filter/UWB sensor 10Hz/UWB noise at 10 Hz/UWB-like noise d4 ==
  Gain : Gain  Gain=0.75
  Gain1 : Gain  Gain=AMPd4
  LTI System1 : cstblocks/LTI System  sys=c2d(tf(1,[0.75 1])*tf([3000 0],[3000 1]),1/10)  IC=[]  PadeOrder=0
  Random Number : RandomNumber  Variance=0.01  Seed=13  SampleTime=1/freq_UWB
  d4_err : Outport
  wires:
  Gain1/1 -> Gain/1
  Gain/1 -> LTI System1/1
  Random Number/1 -> Gain1/1
  LTI System1/1 -> d4_err/1

== system navigation_filter/UWB sensor 10Hz/UWB noise at 10 Hz/UWB-like noise d5 ==
  Gain : Gain  Gain=0.75
  Gain1 : Gain  Gain=AMPd4
  LTI System1 : cstblocks/LTI System  sys=c2d(tf(1,[0.75 1])*tf([3000 0],[3000 1]),1/10)  IC=[]  PadeOrder=0
  Random Number : RandomNumber  Variance=0.01  Seed=13  SampleTime=1/freq_UWB
  d4_err : Outport
  wires:
  Gain1/1 -> Gain/1
  Gain/1 -> LTI System1/1
  Random Number/1 -> Gain1/1
  LTI System1/1 -> d4_err/1

== system navigation_filter/UWB sensor 10Hz/UWB noise at 10 Hz/UWB-like noise d6 ==
  Gain : Gain  Gain=0.75
  Gain1 : Gain  Gain=AMPd4
  LTI System1 : cstblocks/LTI System  sys=c2d(tf(1,[0.75 1])*tf([3000 0],[3000 1]),1/10)  IC=[]  PadeOrder=0
  Random Number : RandomNumber  Variance=0.01  Seed=13  SampleTime=1/freq_UWB
  d4_err : Outport
  wires:
  Gain1/1 -> Gain/1
  Gain/1 -> LTI System1/1
  Random Number/1 -> Gain1/1
  LTI System1/1 -> d4_err/1

== system navigation_filter/UWB sensor 10Hz/UWB noise at 10 Hz/UWB-like noise d7 ==
  Gain : Gain  Gain=0.75
  Gain1 : Gain  Gain=AMPd4
  LTI System1 : cstblocks/LTI System  sys=c2d(tf(1,[0.75 1])*tf([3000 0],[3000 1]),1/10)  IC=[]  PadeOrder=0
  Random Number : RandomNumber  Variance=0.01  Seed=13  SampleTime=1/freq_UWB
  d4_err : Outport
  wires:
  Gain1/1 -> Gain/1
  Gain/1 -> LTI System1/1
  Random Number/1 -> Gain1/1
  LTI System1/1 -> d4_err/1

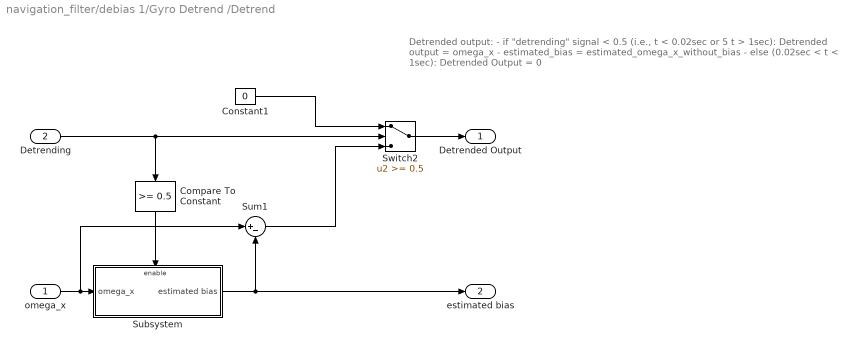
== system navigation_filter/debias 1/Gyro Detrend /Detrend ==
  note: Detrended output:
      | - if "detrending" signal < 0.5 (i.e., t < 0.02sec or 5 t > 1sec): Detrended output = omega_x - estimated_bias = estimated_omega_x_without_bias
      | - else (0.02sec < t < 1sec):  Detrended Output = 0
  omega_x : Inport
  Detrending : Inport  Port=2
  Compare To Constant : simulink/Logic and Bit Operations/Compare To Constant  relop=>=  const=0.5  OutDataTypeStr=boolean
  Constant1 : Constant  Value=0  OutDataTypeStr=single
  Subsystem : Subsystem  TreatAsAtomicUnit=on
  Sum1 : Sum  Inputs=|+-  InputSameDT=on  SaturateOnIntegerOverflow=on  OutDataTypeStr=Inherit: Same as first input
  Switch2 : Switch  Threshold=0.5
  Detrended Output : Outport
  "estimated bias " : Outport  Port=2
  wires:
  Subsystem/1("estimated bias ") -> Sum1/2, "estimated bias "/1
  Compare To Constant/1 -> Subsystem/Enable
  Sum1/1 -> Switch2/3
  omega_x/1 -> Subsystem/1(omega_x), Sum1/1
  Constant1/1 -> Switch2/1
  Detrending/1 -> Switch2/2, Compare To Constant/1
  Switch2/1 -> Detrended Output/1

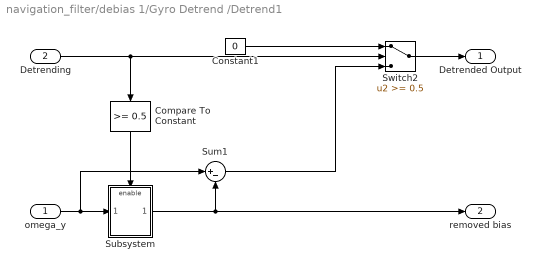
== system navigation_filter/debias 1/Gyro Detrend /Detrend1 ==
  omega_y : Inport
  Detrending : Inport  Port=2
  Compare To Constant : simulink/Logic and Bit Operations/Compare To Constant  relop=>=  const=0.5  OutDataTypeStr=boolean
  Constant1 : Constant  Value=0  OutDataTypeStr=single
  Subsystem : Subsystem  TreatAsAtomicUnit=on
  Sum1 : Sum  Inputs=|+-  InputSameDT=on  SaturateOnIntegerOverflow=on  OutDataTypeStr=Inherit: Same as first input
  Switch2 : Switch  Threshold=0.5
  Detrended Output : Outport
  "removed bias " : Outport  Port=2
  wires:
  Switch2/1 -> Detrended Output/1
  Detrending/1 -> Switch2/2, Compare To Constant/1
  Constant1/1 -> Switch2/1
  omega_y/1 -> Sum1/1, Subsystem/1(acc_y)
  Sum1/1 -> Switch2/3
  Compare To Constant/1 -> Subsystem/Enable
  Subsystem/1("removed bias ") -> Sum1/2, "removed bias "/1

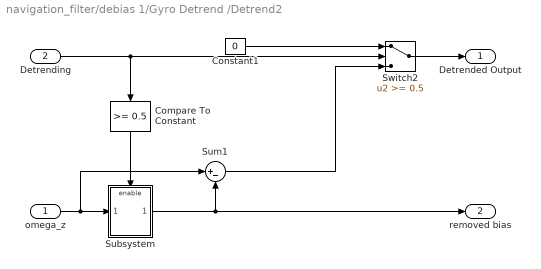
== system navigation_filter/debias 1/Gyro Detrend /Detrend2 ==
  omega_z : Inport
  Detrending : Inport  Port=2
  Compare To Constant : simulink/Logic and Bit Operations/Compare To Constant  relop=>=  const=0.5  OutDataTypeStr=boolean
  Constant1 : Constant  Value=0  OutDataTypeStr=single
  Subsystem : Subsystem  TreatAsAtomicUnit=on
  Sum1 : Sum  Inputs=|+-  InputSameDT=on  SaturateOnIntegerOverflow=on  OutDataTypeStr=Inherit: Same as first input
  Switch2 : Switch  Threshold=0.5
  Detrended Output : Outport
  "removed bias " : Outport  Port=2
  wires:
  Switch2/1 -> Detrended Output/1
  Detrending/1 -> Switch2/2, Compare To Constant/1
  Constant1/1 -> Switch2/1
  omega_z/1 -> Sum1/1, Subsystem/1(acc_y)
  Sum1/1 -> Switch2/3
  Compare To Constant/1 -> Subsystem/Enable
  Subsystem/1("removed bias ") -> Sum1/2, "removed bias "/1

== system navigation_filter/debias 1/Gyro Detrend /Detrend/Subsystem ==
  note: Spiegazione di questo subsystem:
      |
      | Questo fa la media di omega_x nel tempo. Infatti, nei primi 0.5sec la omega_x vale 0 + bias + noise. Facendo la media nel tempo, il white noise si annulla (è a media nulla), e così il valore medio è uguale al bias.
      | Quando enable = 0 (i.e., per t >= 0.5 sec) il subsystem mantiene costante l'ultimo valore in uscita
  omega_x : Inport
  Enable : EnablePort
  Constant : Constant  OutDataTypeStr=single
  Discrete-Time Integrator : DiscreteIntegrator  SampleTime=ST  ICPrevOutput=DiscIntNeverNeededParam  ICPrevScaledInput=DiscIntNeverNeededParam
  Discrete-Time Integrator1 : DiscreteIntegrator  InitialCondition=eps  SampleTime=ST  ICPrevOutput=DiscIntNeverNeededParam  ICPrevScaledInput=DiscIntNeverNeededParam
  Product1 : Product  Inputs=*/  InputSameDT=on  RndMeth=Zero  SaturateOnIntegerOverflow=on  OutDataTypeStr=Inherit: Same as first input
  Scope : Scope  NumInputPorts=2
  "estimated bias " : Outport
  wires:
  omega_x/1 -> Discrete-Time Integrator/1, Scope/1
  Discrete-Time Integrator/1 -> Product1/1
  Product1/1 -> "estimated bias "/1, Scope/2
  Discrete-Time Integrator1/1 -> Product1/2
  Constant/1 -> Discrete-Time Integrator1/1

== system navigation_filter/debias 1/Gyro Detrend /Detrend1/Subsystem ==
  acc_y : Inport
  Enable : EnablePort
  Constant : Constant  OutDataTypeStr=single
  Discrete-Time Integrator : DiscreteIntegrator  SampleTime=ST  ICPrevOutput=DiscIntNeverNeededParam  ICPrevScaledInput=DiscIntNeverNeededParam
  Discrete-Time Integrator1 : DiscreteIntegrator  InitialCondition=eps  SampleTime=ST  ICPrevOutput=DiscIntNeverNeededParam  ICPrevScaledInput=DiscIntNeverNeededParam
  Product1 : Product  Inputs=*/  InputSameDT=on  RndMeth=Zero  SaturateOnIntegerOverflow=on  OutDataTypeStr=Inherit: Same as first input
  "removed bias " : Outport
  wires:
  Constant/1 -> Discrete-Time Integrator1/1
  Discrete-Time Integrator1/1 -> Product1/2
  Product1/1 -> "removed bias "/1
  Discrete-Time Integrator/1 -> Product1/1
  acc_y/1 -> Discrete-Time Integrator/1

== system navigation_filter/debias 1/Gyro Detrend /Detrend2/Subsystem ==
  acc_y : Inport
  Enable : EnablePort
  Constant : Constant  OutDataTypeStr=single
  Discrete-Time Integrator : DiscreteIntegrator  SampleTime=ST  ICPrevOutput=DiscIntNeverNeededParam  ICPrevScaledInput=DiscIntNeverNeededParam
  Discrete-Time Integrator1 : DiscreteIntegrator  InitialCondition=eps  SampleTime=ST  ICPrevOutput=DiscIntNeverNeededParam  ICPrevScaledInput=DiscIntNeverNeededParam
  Product1 : Product  Inputs=*/  InputSameDT=on  RndMeth=Zero  SaturateOnIntegerOverflow=on  OutDataTypeStr=Inherit: Same as first input
  "removed bias " : Outport
  wires:
  Constant/1 -> Discrete-Time Integrator1/1
  Discrete-Time Integrator1/1 -> Product1/2
  Product1/1 -> "removed bias "/1
  Discrete-Time Integrator/1 -> Product1/1
  acc_y/1 -> Discrete-Time Integrator/1

== matlab function navigation_filter/q2eul ==
  data: u input; y output
function y = fcn(u)
    y = quat2eul(u,"ZYX");
    y = rad2deg(y);

== matlab function navigation_filter/MATLAB Function1 ==
  data: q input; euler output
function euler = quat2euler(q)

% quat2euler Convert quaternion to Euler angles (roll, pitch, yaw)
% Input:  
%   q - quaternion as a 1x4 vector [w x y z] or Nx4 matrix
% Output: 
%   euler - Nx3 matrix of Euler angles [roll pitch yaw] in radians

    if size(q, 2) ~= 4
        error('Quaternion must be a Nx4 matrix: [w x y z]');
    end

    % Normalize quaternion
    q = q ./ vecnorm(q, 2, 2);

    w = q(:,1);
    x = q(:,2);
    y = q(:,3);
    z = q(:,4);

    % Compute Euler angles
    roll  = atan2(2*(w.*x + y.*z), 1 - 2*(x.^2 + y.^2));
    pitch = asin(2*(w.*y - z.*x));
    yaw   = atan2(2*(w.*z + x.*y), 1 - 2*(y.^2 + z.^2));

    euler = [roll, pitch, yaw];
end

== matlab function navigation_filter/Filter_attitute ==
  data: mag_meas input; x_out output; omega_meas input; Q parameter; dt parameter
function x_out = filter_attitude(mag_meas, omega_meas, Q, dt)
    %% definition of variables
    % state vector - [q(4), omega(3), gyro_bias(3)] -> 10-dim

    persistent P % covariance matrix 
    persistent x 

    %% Initialization
    if isempty(P)   % this is done in the first cycle --> the persistent variables are inititialized
        P = 10*Q;
        P(8:10,8:10) = P(8:10,8:10)*10^5; % apriori esteem of velocity are bad
        
        x = single(zeros(10,1));
        x(1) = 1; % element of the quaternion q_w = 1
        x(5:7) = omega_meas;
    end

    %% Prediction
    [x, P] = prediction(x, dt, Q, P);

    %% Correction

    %%
    x_out = x;
end



function [x, P] = prediction(x, dt, Q, P)
% update the predicted state
    qw = x(1); qx = x(2); qy = x(3); qz = x(4);         % quaternion (from nav to body)
    w_x = x(5); w_y = x(6); w_z = x(7);                 % omega (body frame)
    byas_gx = x(8); byas_gy = x(9); byas_gz = x(10);    % byass gyro

    % % attitude - quaternion update
    % q0 = quaternion(qw, qx, qy, qz);
    % d_ang = [w_x; w_y; w_z] .* dt;  % delta angle (euler) 
    % %d_q = eul2quat([d_ang(3), d_ang(2), d_ang(1)]);  % delta angle (quaternion)
    % d_q = quaternion([d_ang(3), d_ang(2), d_ang(1)], 'eulerd', 'ZYX', 'frame'); 
    
    % attitude - quaternion update
    q0 = quaternion(qw, qx, qy, qz);
    d_ang = [w_x; w_y; w_z] .* dt;  % delta angle (euler) 
    %d_q = eul2quat([d_ang(3), d_ang(2), d_ang(1)]);  % delta angle (quaternion)
    d_q = quaternion([d_ang(3), d_ang(2), d_ang(1)], 'eulerd', 'ZYX', 'frame'); 
    new_quat = q0*d_q; %q_multi([qw,qx,qy,qz],d_q);

    % output:
    x = [compact(new_quat), w_x, w_y, w_z, byas_gx, byas_gy, byas_gz]';

    % P
    % F = single(F_matrix(north,east,down,vel_n,vel_e,vel_d,acc_x,acc_y,acc_z,q_w,q_x,q_y,q_z,w_x,w_y,w_z,byas_gx,byas_gy,byas_gz,dt));
    % P = F*P*F' + Q;
    P = 10*Q;
    
end

function [x, P] = correction(x, P, measure, sensor_covariances, fuse)

end

== matlab function navigation_filter/MATLAB Function3 ==
  data: q input; euler output
function euler = quat2euler(q)
% quat2euler Convert quaternion to Euler angles (roll, pitch, yaw)
% Input:  
%   q - quaternion as a 1x4 vector [w x y z] or Nx4 matrix
% Output: 
%   euler - Nx3 matrix of Euler angles [roll pitch yaw] in radians

    if size(q, 2) ~= 4
        error('Quaternion must be a Nx4 matrix: [w x y z]');
    end

    % Normalize quaternion
    q = q ./ vecnorm(q, 2, 2);

    w = q(:,1);
    x = q(:,2);
    y = q(:,3);
    z = q(:,4);

    % Compute Euler angles
    roll  = atan2(2*(w.*x + y.*z), 1 - 2*(x.^2 + y.^2));
    pitch = asin(2*(w.*y - z.*x));
    yaw   = atan2(2*(w.*z + x.*y), 1 - 2*(y.^2 + z.^2));

    euler = [roll, pitch, yaw];
end

== matlab function navigation_filter/MATLAB Function2 ==
  data: q_c input; eulerAngles output
function eulerAngles = quaternion2euler(q_c)
%QUATERNION2EULER Converts quaternion to Euler angles [yaw, pitch, roll]
% Input:
%   q_c = [qw, qx, qy, qz] - a quaternion (4x1)
% Output:
%   eulerAngles - [yaw, pitch, roll] in radians (ZYX rotation order)

    q = quaternion(q_c');

    % Ensure quaternion is normalized
    q = normalize(q);

    % Convert to Euler angles using ZYX convention (yaw-pitch-roll)
    eulerAngles = eulerd(q, 'ZYX', 'frame');

    % % Convert degrees to radians
    % eulerAngles = deg2rad(eulerAngles);
    
    % Return as [yaw, pitch, roll]
    eulerAngles = eulerAngles(:)'; % ensure row vector
end

== matlab function navigation_filter/q2eul_ ==
  data: u input; y output
function y = fcn(u)
    y = quat2eul(u,"ZYX");
    y = rad2deg(y);
